simulink model "rpiHROtest06"  (R2016a)
settings: Solver=VariableStepAuto  StartTime=0.0  StopTime=inf  RelTol=1e-3
libraries: dsparch4 x3, embdlinuxlib x2, dspmlti4 x1, dspvision x1, simulink x1, sdrrlib x1
settings Model: Creator=yfujii  LastModifiedBy=yfujii

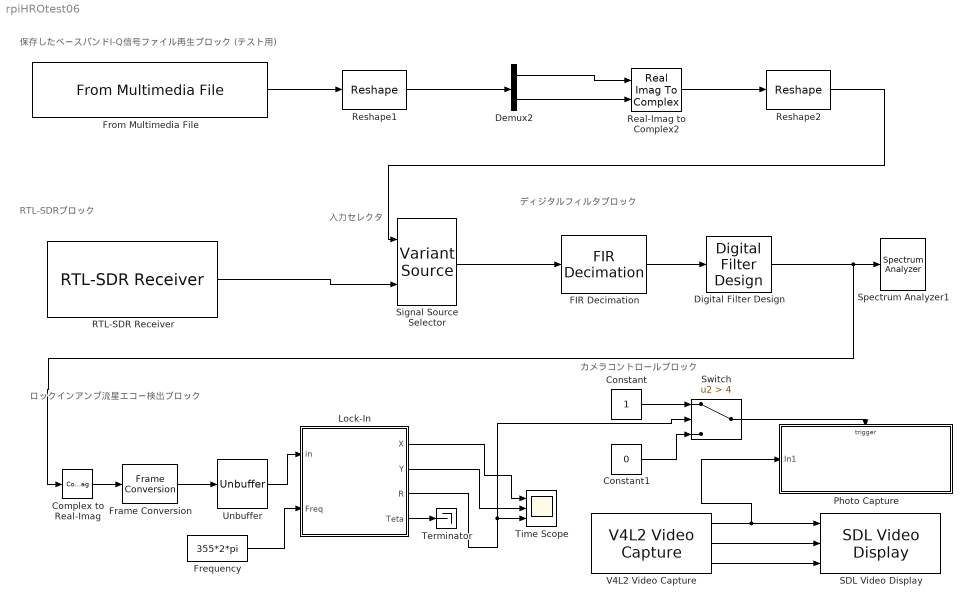
== system rpiHROtest06 ==
  note: ディジタルフィルタブロック
  note: 保存したベースバンドI-Q信号ファイル再生ブロック (テスト用)
  note: RTL-SDRブロック
  note: カメラコントロールブロック
  note: ロックインアンプ流星エコー検出ブロック
  note: 入力セレクタ
  Complex to Real-Imag : ComplexToRealImag  Output=Real
  Constant : Constant
  Constant1 : Constant  Value=0
  Demux2 : Demux  Outputs=[1024, -1]
  Digital Filter Design : dsparch4/Digital Filter Design  mwdsp_browser_bugfix_var=off
  FIR Decimation : dspmlti4/FIR Decimation  FilterSource=Dialog parameters  h=fir1(100, 0.005)  D=50  filtStruct=Direct form  FilterObject=FDECIM  InputProcessing=Columns as channels (frame based)  framing=Allow multirate processing  inputOffset=0  outputBufInitCond=0  roundingMode=Floor  overflowMode=off  firstCoeffDataTypeStr=Inherit: Same word length as input  firstCoeffMin=[]  firstCoeffMax=[]  firstCoeffLastDataTypeStr=Inherit: Same word length as input  outputDataTypeStr=Inherit: Same as accumulator  outputMin=[]  outputMax=[]  outputLastDataTypeStr=Inherit: Same as accumulator
  Frame Conversion : FrameConversion  InheritSamplingMode=off  OutFrame=Sample-based
  Frequency : Constant  Value=355*2*pi
  From Multimedia File : dspvision/From Multimedia File  inputFilename=C:\Users\yfujii\Documents\bitbucket\rpiHROcamera\SDRSharp_20160813_065105Z_53751kHz_IQ.wav  loop=on  numPlays=inf  outputStreams=Audio only  videoDataType=single  audioDataType=double  inheritSampleTime=on  userDefinedSampleTime=1/30  noAudioOutput=off  isIntensityVideo=off  fourcc=RGB  colorVideoFormat=Separate color signals  outputEOF=off  dataOrg=Column-major  audioFrameSize=1024  computeAudioFrameSize=off  outSamplingMode=Sample based
  Lock-In : Subsystem  Description=Lock in Amplifier  mask{freq=357*2*pi, harmonic=1, order=2, pass=5}
      mask prompts: freq "Detection frequency (rad/sec)"; order "FilterOrder"; pass "Pass band edge frequency"
      mask help:
      | LOCK-IN AMPLIFIER
      | Copyright (c) Predrag Drljaca 2002
      | Choose internal frequency of the clock generator, harminic of the signal you want to measure, as well as the order and the frequency of the internal low pass filter.
      mask Display:
      | plot([1 40 40 60 60 90], [3 3 50 50 3 3]);
      | text(7,60,'Lock-in ampli');
      | plot([0 1], [65 65]);
  Photo Capture : Subsystem
  RTL-SDR Receiver : sdrrlib/RTL-SDR Receiver  SourceLibraryInfo="This block requires <a href=\"http://www.mathworks.com/hardware-support/rtl-sdr.html\">Communications System Toolbox Support Package for RTL-SDR Radio</a>"  sobjType=sdrr.internal.SDRRTLReceiverSL  IPAddress=0  dataUDPPort=-1  ctrlUDPPort=-1  subDeviceList=nosubdev  sdrBlockType=SDRBlockTypeSLT.SDRRxBlock  requester=UNUSED_BY_SFCN  sdrExecutionMode=SDRExecutionModeSLT.ExecModeHW  LostSamplesOutputPort=off  OutputDataType=int16  FrameLength=1024  EnableBurstMode=off  NumFramesInBurst=20  BypassUserLogic=off  DecimatorSelect=DDC decimator  SourceSelect=RF data  SineAmplitude=16000  EnableInternalClock=off  BypassIQBalance=off  CenterFrequency=102.5e6  IFBandwidth=40e6  ADCRateSource=Dialog  ADCRate=250e3  CenterFrequencySource=Dialog  GainSource=AGC  IntermediateFrequency=0  Gain=0  DecimationFactorSource=Dialog  DecimationFactor=512  RFFrequencyIsTunable=logical(0)  SampleTime=(1024)/(250e3)  IFBandwidthSource=Dialog  SineFrequency=30000  BypassDCBlockingFilter=off  IntermediateFrequencySource=Dialog  IQBalanceCoefficients=64  SkipAllHardwareResetAndInitialization=off  EnableIQCalibrationTable=on  CacheIQCalibrationTable=off  EnableOffsetTuning=off  EnableRTLAGC=off  EnableTestMode=off  EnableTunerAGC=on  FrequencyCorrectionSource=Dialog  FrequencyCorrection=0  NumMLBuffers=128  NumUSBBuffers=16  LatencyOutputPort=off  RTLCrystalFrequency=28800000  TunerCrystalFrequency=28800000
  Real-Imag to Complex2 : RealImagToComplex
  Reshape1 : Reshape  OutputDimensionality=Row vector (2-D)  OutputDimensions=[1]
  Reshape2 : Reshape  OutputDimensionality=Column vector (2-D)  OutputDimensions=[1]
  SDL Video Display : embdlinuxlib/SDL Video Display  pixelFormat=YCbCr 4:2:2  pixelOrder=Planar  rowMajor=on  blockPlatform=Raspberry Pi
  Signal Source Selector : VariantSource  OverrideUsingVariant=ReadFromFile  mask(Signal Source Selector){sigSource=Captured Signal}
      mask prompts: sigSource "Signal source:"
      mask help: Select one of the connected sources as the signal source for this example.
      mask TypeOptions sigSource: Captured Signal | RTL-SDR Radio
      mask Callback sigSource:
      | if strcmp(get_param(gcb, 'sigSource'), 'Captured Signal')
      |   set_param(gcb, 'OverrideUsingVariant', 'ReadFromFile')
      | elseif strcmp(get_param(gcb, 'sigSource'), 'RTL-SDR Radio')
      |   set_param(gcb, 'OverrideUsingVariant', 'RTLSDRRadio')
      | end
  Spectrum Analyzer1 : SpectrumAnalyzer
  Switch : Switch  Criteria=u2 > Threshold  Threshold=4
  Terminator : Terminator
  Time Scope : Scope  NumInputPorts=3
  Unbuffer : Unbuffer  SampleBasedProcessing=Same as frame based
  V4L2 Video Capture : embdlinuxlib/V4L2 Video Capture  m_devName='/dev/video0'  roi=[0, 0, 640, 480]  imSizeSelection=320x240  imSize=[640, 480]  pixelFormat=YCbCr 4:2:2  pixelOrder=Planar  sampleTime=1/10  simOutput=Colorbars  blockPlatform=Raspberry Pi
  wires:
  FIR Decimation/1 -> Digital Filter Design/1
  Digital Filter Design/1 -> Spectrum Analyzer1/1, Complex to Real-Imag/1
  From Multimedia File/1 -> Reshape1/1
  Demux2/1 -> Real-Imag to Complex2/1
  Reshape1/1 -> Demux2/1
  Demux2/2 -> Real-Imag to Complex2/2
  Real-Imag to Complex2/1 -> Reshape2/1
  RTL-SDR Receiver/1 -> Signal Source Selector/2
  V4L2 Video Capture/1 -> Photo Capture/1(In1), SDL Video Display/1
  V4L2 Video Capture/2 -> SDL Video Display/2
  V4L2 Video Capture/3 -> SDL Video Display/3
  Lock-In/3(R) -> Time Scope/3, Switch/2
  Constant/1 -> Switch/1
  Constant1/1 -> Switch/3
  Switch/1 -> Photo Capture/Trigger
  Reshape2/1 -> Signal Source Selector/1
  Lock-In/4(Teta) -> Terminator/1
  Lock-In/2(Y) -> Time Scope/2
  Signal Source Selector/1 -> FIR Decimation/1
  Lock-In/1(X) -> Time Scope/1
  Frame Conversion/1 -> Unbuffer/1
  Unbuffer/1 -> Lock-In/1(in)
  Complex to Real-Imag/1 -> Frame Conversion/1
  Frequency/1 -> Lock-In/2(Freq)

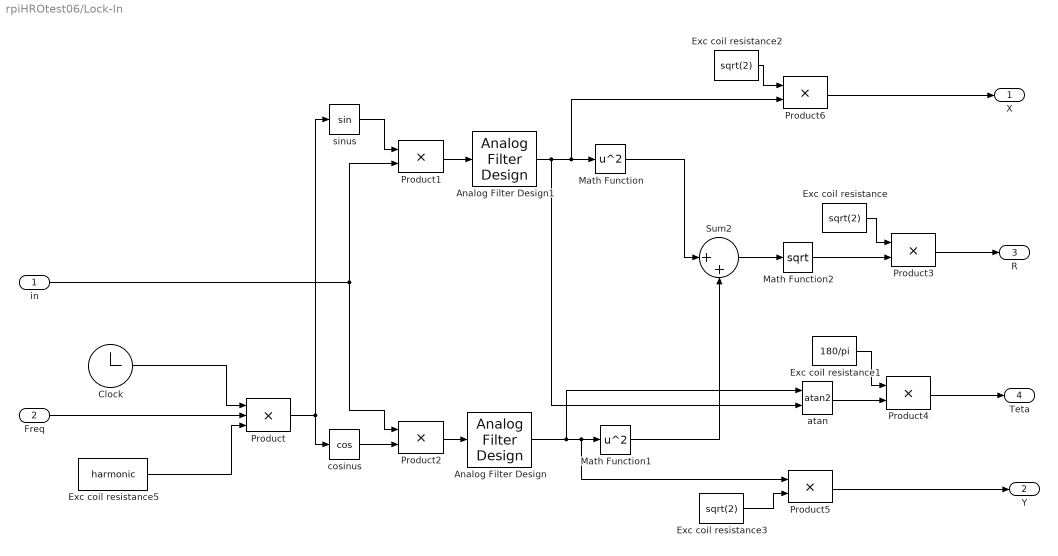
== system rpiHROtest06/Lock-In ==
  in : Inport
  Freq : Inport  Port=2
  Analog Filter Design : dsparch4/Analog Filter Design  method=Butterworth  filttype=Lowpass  N=order  Wlo=pass  Whi=80  Rp=2  Rs=40
  Analog Filter Design1 : dsparch4/Analog Filter Design  method=Butterworth  filttype=Lowpass  N=order  Wlo=pass  Whi=80  Rp=2  Rs=40
  Clock : Clock
  Exc coil resistance : Constant  Value=sqrt(2)
  Exc coil resistance1 : Constant  Value=180/pi
  Exc coil resistance2 : Constant  Value=sqrt(2)
  Exc coil resistance3 : Constant  Value=sqrt(2)
  Exc coil resistance5 : Constant  Value=harmonic
  Math Function : Math  Operator=square  SaturateOnIntegerOverflow=on
  Math Function1 : Math  Operator=square  SaturateOnIntegerOverflow=on
  Math Function2 : Math  Operator=sqrt  SaturateOnIntegerOverflow=on
  Product : Product  Inputs=***  SaturateOnIntegerOverflow=on  RndMeth=Zero  InputSameDT=on  OutDataTypeStr=Inherit: Same as first input
  Product{1..6} (6 alike) : Product  SaturateOnIntegerOverflow=on  RndMeth=Zero  InputSameDT=on  OutDataTypeStr=Inherit: Same as first input
  Sum2 : Sum  Inputs=|++  SaturateOnIntegerOverflow=on  InputSameDT=on  OutDataTypeStr=Inherit: Same as first input
  atan : Trigonometry  Operator=atan2  OutputSignalType=real
  cosinus : Trigonometry  Operator=cos
  sinus : Trigonometry
  X : Outport
  Y : Outport  Port=2
  R : Outport  Port=3
  Teta : Outport  Port=4
  wires:
  Product5/1 -> Y/1
  Product1/1 -> Analog Filter Design1/1
  Product2/1 -> Analog Filter Design/1
  Exc coil resistance2/1 -> Product6/1
  Product6/1 -> X/1
  Exc coil resistance3/1 -> Product5/2
  Math Function1/1 -> Sum2/2
  Analog Filter Design/1 -> Product5/1, Math Function1/1, atan/1
  Math Function/1 -> Sum2/1
  Analog Filter Design1/1 -> Product6/2, Math Function/1, atan/2
  Exc coil resistance1/1 -> Product4/1
  Product4/1 -> Teta/1
  atan/1 -> Product4/2
  Exc coil resistance/1 -> Product3/1
  Product3/1 -> R/1
  Math Function2/1 -> Product3/2
  Sum2/1 -> Math Function2/1
  cosinus/1 -> Product2/2
  in/1 -> Product2/1, Product1/2
  sinus/1 -> Product1/1
  Freq/1 -> Product/2
  Product/1 -> sinus/1, cosinus/1
  Clock/1 -> Product/1
  Exc coil resistance5/1 -> Product/3

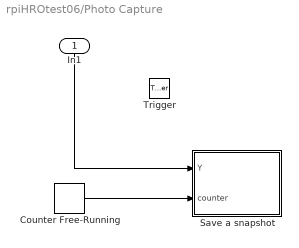
== system rpiHROtest06/Photo Capture ==
  In1 : Inport
  Trigger : TriggerPort  VariantControl=Variant
  Counter Free-Running : simulink/Sources/Counter Free-Running  NumBits=32  tsamp=-1
  Save a snapshot : MATLAB Function  TreatAsAtomicUnit=on
  wires:
  In1/1 -> Save a snapshot/1(Y)
  Counter Free-Running/1 -> Save a snapshot/2(counter)

== matlab function rpiHROtest06/Photo Capture/Save a snapshot ==
  data: Y input; counter input
function fcn(Y, counter)
%#codegen

% Save 160x120 grayscale image to a file
format = ['%d ', 0];
fname  = coder.nullcopy(uint8(zeros(1, 32)));
coder.ceval('sprintf', coder.wref(fname), ['img%d.dat', 0], counter);
fd = coder.opaque('FILE *');
fd = coder.ceval('fopen', fname, ['w', 0]);
for i = 1:160
    for j = 1:120
        coder.ceval('fprintf', fd, format, Y(i, j));
    end
end
coder.ceval('fclose', fd);
